simulink model "link_subsystem_test"  (Simulink 8.4)
settings: Solver=ode45  StartTime=0.0  StopTime=10.0  RelTol=1e-3
libraries: link_subsystem_lib_test x2
settings Model: Creator=arnaud  LastModifiedBy=arnaud
settings DataIOCC: SaveFormat=Structure  SignalLoggingSaveFormat=Dataset  SaveOutput=off  SaveTime=off
settings OptimizationCC: ExpressionDepthLimit=128
settings DebuggingCC: UnderspecifiedInitializationDetection=Simplified  MergeDetectMultiDrivingBlocksExec=error  FcnCallInpInsideContextMsg=EnableAllAsError  StateNameClashWarn=none
settings GRTTargetCC: CombineOutputUpdateFcns=on  GRTInterface=off

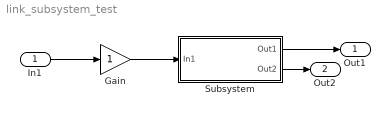
== system link_subsystem_test ==
  In1 : Inport  OutDataTypeStr=double  PortDimensions=1  SampleTime=0
  Gain : Gain
  Subsystem : Subsystem  TreatAsAtomicUnit=on
  Out1 : Outport  OutDataTypeStr=double  PortDimensions=1  SampleTime=0
  Out2 : Outport  Port=2  OutDataTypeStr=double  PortDimensions=1  SampleTime=0
  wires:
  In1/1 -> Gain/1
  Subsystem/1(Out1) -> Out1/1
  Gain/1 -> Subsystem/1(In1)
  Subsystem/2(Out2) -> Out2/1

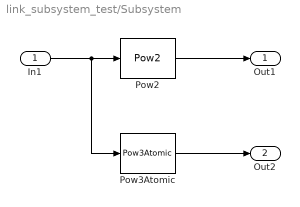
== system link_subsystem_test/Subsystem ==
  In1 : Inport
  Pow2 : link_subsystem_lib_test/Pow2
  Pow3Atomic : link_subsystem_lib_test/Pow3Atomic
  Out1 : Outport
  Out2 : Outport  Port=2
  wires:
  In1/1 -> Pow3Atomic/1, Pow2/1
  Pow2/1 -> Out1/1
  Pow3Atomic/1 -> Out2/1
